simulink model "AutoDriveSystemDemo"  (R2022a)
settings: Solver=ode5  StartTime=0.0  StopTime=10000  FixedStep=.0001  RelTol=1e-3  AbsTol=1e-6
settings Model: FPTRunName=Active  ExtModeTrigMode=oneshot  ExtModeArmWhenConnect=off  Creator=The MathWorks, Inc.  LastModifiedBy=Antonio Alonso
settings SolverCC: AutoScaleAbsTol=off  AlgebraicLoopSolver=TrustRegion
settings DataIOCC: ExternalInput=runHot, vCar, lidarData, objectClassification  LoadExternalInput=on  SaveFormat=Array  SaveOutput=off  SaveTime=off  ReturnWorkspaceOutputs=off
settings OptimizationCC: BooleanDataType=off  ExpressionDepthLimit=2147483647  InitFltsAndDblsToZero=on  EfficientMapNaN2IntZero=off  LifeSpan=inf  BufferReusableBoundary=off
settings DebuggingCC: SaveWithParameterizedLinksMsg=none  UnderspecifiedInitializationDetection=Classic  MergeDetectMultiDrivingBlocksExec=none  SignalResolutionControl=TryResolveAllWithWarning  MultiTaskDSMMsg=warning  MultiTaskCondExecSysMsg=none  IntegerOverflowMsg=none  FcnCallInpInsideContextMsg=warning  UnconnectedInputMsg=warning  UnconnectedOutputMsg=warning  UnconnectedLineMsg=warning  StateNameClashWarn=warning  SFUnexpectedBacktrackingDiag=warning  SFNoUnconditionalDefaultTransitionDiag=warning  SFExecutionAtInitializationDiag=none  SFMachineParentedDataDiag=warning  IntegerSaturationMsg=none  ArithmeticOperatorsInVariantConditions=warning
settings HardwareCC: ProdBitPerPointer=32  ProdBitPerSizeT=32  ProdBitPerPtrDiffT=32  ProdLargestAtomicFloat=None  ProdIntDivRoundTo=Undefined  ProdEndianess=Unspecified  ProdWordSize=32  ProdHWDeviceType=32-bit Generic  TargetUnknown=on
settings ModelReferenceCC: PropagateSignalLabelsOutOfModel=off
settings SFSimCC: SimUseLocalCustomCode=off  SimParseCustomCode=off  CustomCodeUndefinedFunction=UseInterfaceOnly
settings RTWCC: TemplateMakefile=grt_vc.tmf  RTWUseLocalCustomCode=off
settings CodeAppCC: StateflowObjectComments=on
settings GRTTargetCC: TargetFcnLib=ansi_tfl_tmw.mat  TargetLangStandard=C89/C90 (ANSI)  CombineOutputUpdateFcns=off  GRTInterface=on
settings ConfigComp: CovMetricSettings=dcmtr  CovSaveCumulativeToWorkspaceVar=on  CovSaveSingleToWorkspaceVar=on  CovExternalEMLEnable=off  CovSFcnEnable=off

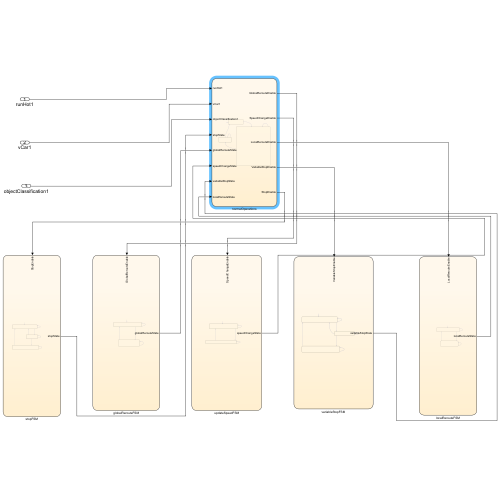
[thumbnail: Simulink's stored preview of the top-level diagram]
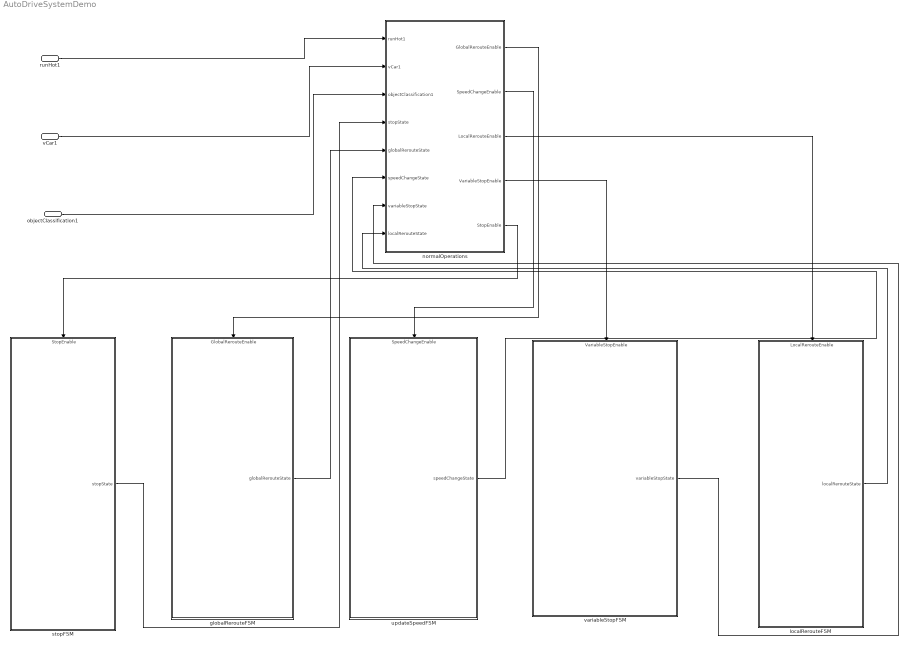
== system AutoDriveSystemDemo ==
  runHot1 : Inport
  vCar1 : Inport  Port=2
  objectClassification1 : Inport  Port=3
  globalRerouteFSM : Stateflow chart  TreatAsAtomicUnit=on
      settings: PortSchema="{\"entries\":[{\"content\":{\"sides\":[{\"content\":{\"connectorIds\":[]},\"type\":\"ConnectorPlacement.EquallySpacedRectSide\",\"uuid\":\"70914dc1-c424-4c74-afae-cf22c09490df\"},{\"content\":{\"connectorIds\":[\"Out1\"],\"side\":\"RIGHT\"},\"type\":\"ConnectorPlacement.EquallySpacedRectSide\",\"uuid\":\"e582008e-93f3-40e6-b55b-57d9ba56b53b\"},{\"content\":{\"connectorIds\":[\"In1\"],\"side\":\"TOP\"},\"type\":\"ConnectorPlacement.EquallySpacedRectSide\",\"uuid\":\"6c4278e7-8a86-4c54-8ec8-adc5a5925567\"}]},\"type\":\"ConnectorPlacement.EquallySpacedConnector\",\"uuid\":\"fe4c801d-5d3b-420c-bc38-aa71b437525e\"}],\"packageUris\":[\"http://schema.mathworks.com/mf0/Connector/R2020b\"],\"version\":\"1.0\"}"
  localRerouteFSM : Stateflow chart  TreatAsAtomicUnit=on
      settings: PortSchema="{\"entries\":[{\"content\":{\"sides\":[{\"content\":{\"connectorIds\":[]},\"type\":\"ConnectorPlacement.EquallySpacedRectSide\",\"uuid\":\"70914dc1-c424-4c74-afae-cf22c09490df\"},{\"content\":{\"connectorIds\":[\"Out1\"],\"side\":\"RIGHT\"},\"type\":\"ConnectorPlacement.EquallySpacedRectSide\",\"uuid\":\"e582008e-93f3-40e6-b55b-57d9ba56b53b\"},{\"content\":{\"connectorIds\":[\"In1\"],\"side\":\"TOP\"},\"type\":\"ConnectorPlacement.EquallySpacedRectSide\",\"uuid\":\"6c4278e7-8a86-4c54-8ec8-adc5a5925567\"}]},\"type\":\"ConnectorPlacement.EquallySpacedConnector\",\"uuid\":\"fe4c801d-5d3b-420c-bc38-aa71b437525e\"}],\"packageUris\":[\"http://schema.mathworks.com/mf0/Connector/R2020b\"],\"version\":\"1.0\"}"
  normalOperations : Stateflow chart  TreatAsAtomicUnit=on
  stopFSM : Stateflow chart  TreatAsAtomicUnit=on
      settings: PortSchema="{\"entries\":[{\"content\":{\"sides\":[{\"content\":{\"connectorIds\":[]},\"type\":\"ConnectorPlacement.EquallySpacedRectSide\",\"uuid\":\"1c7e23b1-b9d9-4abd-9f5f-096c00e3ae2e\"},{\"content\":{\"connectorIds\":[\"Out1\"],\"side\":\"RIGHT\"},\"type\":\"ConnectorPlacement.EquallySpacedRectSide\",\"uuid\":\"486f1451-125f-4bd8-a376-433cd7748c33\"},{\"content\":{\"connectorIds\":[\"In1\"],\"side\":\"TOP\"},\"type\":\"ConnectorPlacement.EquallySpacedRectSide\",\"uuid\":\"97f37c01-0db5-4f76-9b11-8af5d6c70636\"}]},\"type\":\"ConnectorPlacement.EquallySpacedConnector\",\"uuid\":\"d50f914d-de3c-42a5-ab35-c087d4fb0f09\"}],\"packageUris\":[\"http://schema.mathworks.com/mf0/Connector/R2020b\"],\"version\":\"1.0\"}"
  updateSpeedFSM : Stateflow chart  TreatAsAtomicUnit=on
      settings: PortSchema="{\"entries\":[{\"content\":{\"sides\":[{\"content\":{\"connectorIds\":[]},\"type\":\"ConnectorPlacement.EquallySpacedRectSide\",\"uuid\":\"70914dc1-c424-4c74-afae-cf22c09490df\"},{\"content\":{\"connectorIds\":[\"Out1\"],\"side\":\"RIGHT\"},\"type\":\"ConnectorPlacement.EquallySpacedRectSide\",\"uuid\":\"e582008e-93f3-40e6-b55b-57d9ba56b53b\"},{\"content\":{\"connectorIds\":[\"In1\"],\"side\":\"TOP\"},\"type\":\"ConnectorPlacement.EquallySpacedRectSide\",\"uuid\":\"6c4278e7-8a86-4c54-8ec8-adc5a5925567\"}]},\"type\":\"ConnectorPlacement.EquallySpacedConnector\",\"uuid\":\"fe4c801d-5d3b-420c-bc38-aa71b437525e\"}],\"packageUris\":[\"http://schema.mathworks.com/mf0/Connector/R2020b\"],\"version\":\"1.0\"}"
  variableStopFSM : Stateflow chart  TreatAsAtomicUnit=on
      settings: PortSchema="{\"entries\":[{\"content\":{\"sides\":[{\"content\":{\"connectorIds\":[]},\"type\":\"ConnectorPlacement.EquallySpacedRectSide\",\"uuid\":\"70914dc1-c424-4c74-afae-cf22c09490df\"},{\"content\":{\"connectorIds\":[\"Out1\"],\"side\":\"RIGHT\"},\"type\":\"ConnectorPlacement.EquallySpacedRectSide\",\"uuid\":\"e582008e-93f3-40e6-b55b-57d9ba56b53b\"},{\"content\":{\"connectorIds\":[\"In1\"],\"side\":\"TOP\"},\"type\":\"ConnectorPlacement.EquallySpacedRectSide\",\"uuid\":\"6c4278e7-8a86-4c54-8ec8-adc5a5925567\"}]},\"type\":\"ConnectorPlacement.EquallySpacedConnector\",\"uuid\":\"fe4c801d-5d3b-420c-bc38-aa71b437525e\"}],\"packageUris\":[\"http://schema.mathworks.com/mf0/Connector/R2020b\"],\"version\":\"1.0\"}"
  wires:
  objectClassification1/1 -> normalOperations/3(objectClassification1)
  vCar1/1 -> normalOperations/2(vCar1)
  runHot1/1 -> normalOperations/1(runHot1)
  normalOperations/5(StopEnable) -> stopFSM/1(StopEnable)
  normalOperations/1(GlobalRerouteEnable) -> globalRerouteFSM/1(GlobalRerouteEnable)
  normalOperations/2(SpeedChangeEnable) -> updateSpeedFSM/1(SpeedChangeEnable)
  normalOperations/4(VariableStopEnable) -> variableStopFSM/1(VariableStopEnable)
  normalOperations/3(LocalRerouteEnable) -> localRerouteFSM/1(LocalRerouteEnable)
  stopFSM/1(stopState) -> normalOperations/4(stopState)
  globalRerouteFSM/1(globalRerouteState) -> normalOperations/5(globalRerouteState)
  updateSpeedFSM/1(speedChangeState) -> normalOperations/6(speedChangeState)
  variableStopFSM/1(variableStopState) -> normalOperations/7(variableStopState)
  localRerouteFSM/1(localRerouteState) -> normalOperations/8(localRerouteState)

== stateflow chart AutoDriveSystemDemo/normalOperations ==
  state manual_mode
    en: normalOpState = 0
    en: ActiveObjectList = []
  state autonomous_mode
    %StopSignEnable
    %VariableStopEnable
    %LocalRerouteEnable
    %GlobalRerouteEnable
    %SpeedChangeEnable
    en: normalOpState = 1
    du: updateObstaclesInProjectedOccupancyZones(ActiveObjectList, VWP, ...
    objectClassification)
    %Figure out which machine is needed if any
    du:[StopSignEnable, VariableStopEnable, LocalRerouteEnable, GlobalRerouteEnable, SpeedChangeEnable] = calculate(ActiveObjectList, logical(StopSignEnable, VariableStopEnable, LocalRerouteEnable, GlobalRerouteEnable, SpeedChangeEnable))
    %Update Enables based on State of Machines, this is done to fix DataRaces
    du: [StopSignEnable, VariableStopEnable, LocalRerouteEnable, GlobalRerouteEnable, SpeedChangeEnable] = updateMachineStates(stopState, globalRerouteState, speedChangeState, variableStopState, localRerouteState)
    %Update Flag for Active Machine
    du: SubMachineRunning = StopSignEnable || VariableStopEnable || ...
    LocalRerouteEnable || GlobalRerouteEnable
  state wait_for_stopped
    en: normalOpState = 2
  manual_mode -> autonomous_mode : [runHot == 1 && VWP.length > 0]
  (default) -> manual_mode
  autonomous_mode -> autonomous_mode [order 2]
  wait_for_stopped -> manual_mode [order 1] : [vCar == 0]
      | {runHot = 0}
  wait_for_stopped -> wait_for_stopped [order 2]
  autonomous_mode -> wait_for_stopped [order 1] : [VWP.length == 0]
      | {updateVWP(VWP, distance)}
  data: stopState function_input; globalRerouteState function_input; speedChangeState function_input; variableStopState function_input; localRerouteState function_input; res function_output; ActiveObjectList function_input; previousConditionals function_input; triggers function_output; ActiveObjectList function_input; VWP function_input; objectClassicication function_input; GlobalRerouteEnable output; SpeedChangeEnable output; LocalRerouteEnable output; VariableStopEnable output; runHot1 input; vCar1 input; objectClassification1 input; StopEnable output; stopState input; globalRerouteState input; speedChangeState input; variableStopState input; localRerouteState input
  function res = updateMachineStates(stopState, globalRerouteState, speedChangeState, variableStopState, localRerouteState):
    | function res = updateMachineStates(stopState, globalRerouteState, speedChangeState, variableStopState, localRerouteState) 
    |     disp("updating machines");
    |     res = true(5);
    |     if stopState == Nan
    |         return;
    |     end
    |     
    |     if (stopState == 0)  
    |         res(1) = false;
    |     end
    |     if globalRerouteState == 0 
    |         res(2) = false;
    |     end
    |     if speedChangeState == 0 
    |         res(3) = false;
    |     end
    |     if variableStopState == 0 
    |         res(4) = false;
    |     end
    |     if localRerouteState == 0 
    |         res(5) = false;
    |     end
    |     
    | end
  function triggers = calculate(ActiveObjectList, previousConditionals):
    | function triggers = calculate(ActiveObjectList, previousConditionals)
    |     triggers = false(5);
    |     triggers = or(triggers, previousConditionals);
    |     %StopSignEnable 
    |     %VariableStopEnable 
    |     %LocalRerouteEnable
    |     %GlobalRerouteEnable
    |     %SpeedChangeEnable
    |     curObject = sort(ActiveObjectList);
    |     if curObject == None
    |         disp("curObject is None")
    |     elseif  curObject == stopSign
    |         triggers(1) = true;
    |         triggers(2) = false;
    |         triggers(3) = false;
    |         triggers(4) = false;
    |     elseif curObject == stopLight || RR || movingObstacle
    |         triggers(1) = false;
    |         triggers(2) = true;
    |         triggers(3) = false;
    |         triggers(4) = false;
    |     elseif requiresLocalReroute(curObject)
    |         triggers(1) = false;
    |         triggers(2) = false;
    |         triggers(3) = true;
    |         triggers(4) = false;
    |     else
    |         triggers(1) = false;
    |         triggers(2) = false;
    |         triggers(3) = false;
    |         triggers(4) = true;
    |     end
    |     if SubMachineRunning == false && abs(vCar - LastSeenSpeedLimit) > 0.5
    |         triggers(5) = true;
    |         
    |     end
  function updateObstaclesInProjectedOccupancyZones(ActiveObjectList, VWP, objectClassicication):
    | function updateObstaclesInProjectedOccupancyZones(ActiveObjectList, VWP, objectClassicication)

== stateflow chart AutoDriveSystemDemo/globalRerouteFSM ==
  state wait_for_globalReroute_enable
    en:  globalRerouteState = 0;
  state slow_while_rerouting
    en: globalRerouteState = 1
    du: newVWP = calculateGlobalRoute()
    ex: turnSignalLightOn()
  (default) -> wait_for_globalReroute_enable
  wait_for_globalReroute_enable -> wait_for_globalReroute_enable [order 2]
  slow_while_rerouting -> wait_for_globalReroute_enable [order 1] : [GlobalRerouteEnable == false || newVWP.length > 0]
      | { updateWaypoints(newVWP);
      |   SubMachineRunning = false;
      |   GlobalRerouteEnable = false; }
  wait_for_globalReroute_enable -> slow_while_rerouting [order 1] : [GlobalRerouteEnable == true]
      | {VWP = updateVWP(VWP, stopDistance)}
  slow_while_rerouting -> slow_while_rerouting [order 2]
  data: GlobalRerouteEnable input; globalRerouteState output

== stateflow chart AutoDriveSystemDemo/updateSpeedFSM ==
  state wait_for_speedChange_enable
    en:  speedChangeState = 0;
  state wait_for_correct_speed
    en:  speedChangeState = 1;
  (default) -> wait_for_speedChange_enable
  wait_for_speedChange_enable -> wait_for_speedChange_enable [order 2]
  wait_for_correct_speed -> wait_for_speedChange_enable [order 1] : [SpeedChangeEnable == false || ...
      |   abs(vCar - LastSeenSpeedLimit) < 0.1]
      | { SubMachineRunning = false;
      |   SpeedChangeEnable = false; }
  wait_for_speedChange_enable -> wait_for_correct_speed [order 1] : [SpeedChangeEnable == true]
      | {VWP = updateVehicleSpeed(VWP, LastSeenSpeedLimit)}
  wait_for_correct_speed -> wait_for_correct_speed [order 2]
  data: SpeedChangeEnable input; speedChangeState output

== stateflow chart AutoDriveSystemDemo/stopFSM ==
  state wait_for_stop_enable
    en:  stopState = 0;
  state wait_for_zero_velocity
    en:  stopState = 1;
  state wait_for_stop_duration
    en:  stopState = 2;
    du:  tNow = getCurrentTime();
  (default) -> wait_for_stop_enable
  wait_for_stop_enable -> wait_for_stop_enable [order 2]
  wait_for_stop_duration -> wait_for_stop_enable [order 1] : [StopEnable == false || tNow >= tStop]
      | { SubMachineRunning = false;
      |   StopEnable = false;}
  wait_for_zero_velocity -> wait_for_stop_enable [order 1] : [StopEnable == false]
  wait_for_stop_enable -> wait_for_zero_velocity [order 1] : [StopEnable == true]
      | {VWP = updateVWP(stopDistance,VWP)}
  wait_for_zero_velocity -> wait_for_zero_velocity [order 3]
  wait_for_zero_velocity -> wait_for_stop_duration [order 2] : [vCar == 0]
      | {tStop = stopDuration + getCurrentTime();}
  wait_for_stop_duration -> wait_for_stop_duration [order 2]
  data: StopEnable input; stopState output

== stateflow chart AutoDriveSystemDemo/variableStopFSM ==
  state wait_for_variableStop_enable
    en:  variableStopState = 0;
  state wait_for_zero_velocity
    en:  variableStopState = 1;
  state wait_while_curObstacle_is_present
    en:  variableStopState = 2;
    en: curObstacle = sort(ActiveObjectList)
  (default) -> wait_for_variableStop_enable
  wait_for_variableStop_enable -> wait_for_variableStop_enable [order 1]
  wait_while_curObstacle_is_present -> wait_for_variableStop_enable [order 1] : [VariableStopEnable == false || ...
      |   ~ismember(curObstacle, ActiveObstacleList)]
      | {SubMachineRunning = false;
      | VariableStopEnable = false;}
  wait_for_zero_velocity -> wait_for_variableStop_enable [order 1] : [VariableStopEnable == false]
  wait_for_variableStop_enable -> wait_for_zero_velocity [order 2] : [VariableStopEnable == true]
      | {VWP = updateVWP(VWP, stopDistance)}
  wait_for_zero_velocity -> wait_for_zero_velocity [order 3]
  wait_for_zero_velocity -> wait_while_curObstacle_is_present [order 2] : [vCar == 0]
  wait_while_curObstacle_is_present -> wait_while_curObstacle_is_present [order 2]
  data: VariableStopEnable input; variableStopState output

== stateflow chart AutoDriveSystemDemo/localRerouteFSM ==
  state wait_for_localReroute_enable
    en:  localRerouteState = 0;
  state slow_while_rerouting
    en: localRerouteState = 1
    du: newVWP = calculateLocalRoute()
    ex: turnSignalLightOn()
  (default) -> wait_for_localReroute_enable
  wait_for_localReroute_enable -> wait_for_localReroute_enable [order 2]
  slow_while_rerouting -> wait_for_localReroute_enable [order 1] : [LocalRerouteEnable == false || newVWP.length > 0]
      | { updateWaypoints(newVWP);
      |   SubMachineRunning = false;
      |   LocalRerouteEnable = false; }
  wait_for_localReroute_enable -> slow_while_rerouting [order 1] : [LocalRerouteEnable == true]
      | {VWP = updateVWP(VWP, stopDistance)}
  slow_while_rerouting -> slow_while_rerouting [order 2]
  data: LocalRerouteEnable input; localRerouteState output
